simulink model "EX_opt_1_model"  (R2025b)
settings: Solver=ode4  StartTime=0.0  StopTime=T_SIMULATION  FixedStep=1e-3  RelTol=1e-3
values from neighbouring files (symbols this model uses):
  d = 0.165    [EX_opt_1.m]
  omega = 2    [EX_opt_1.m]    (also in EX_opt_2.m = zeros(size(t)))
  Q_INITIAL = [1;1;0]    [EX_opt_1.m]
  r = 0.03    [EX_opt_1.m]
  v = 0    [EX_opt_1.m]    (also in EX_opt_2.m = zeros(size(t)))
settings Model: Creator=llp  LastModifiedBy=llp

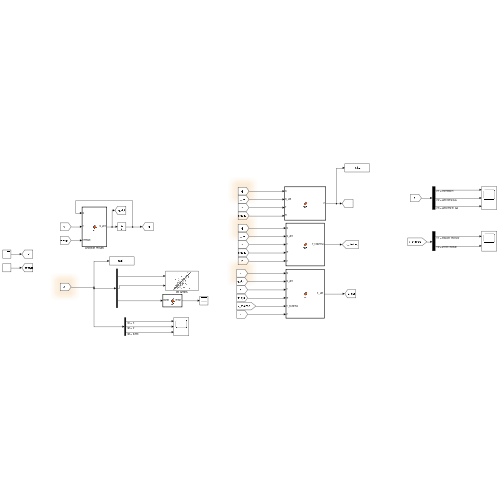
[thumbnail: Simulink's stored preview of the top-level diagram]
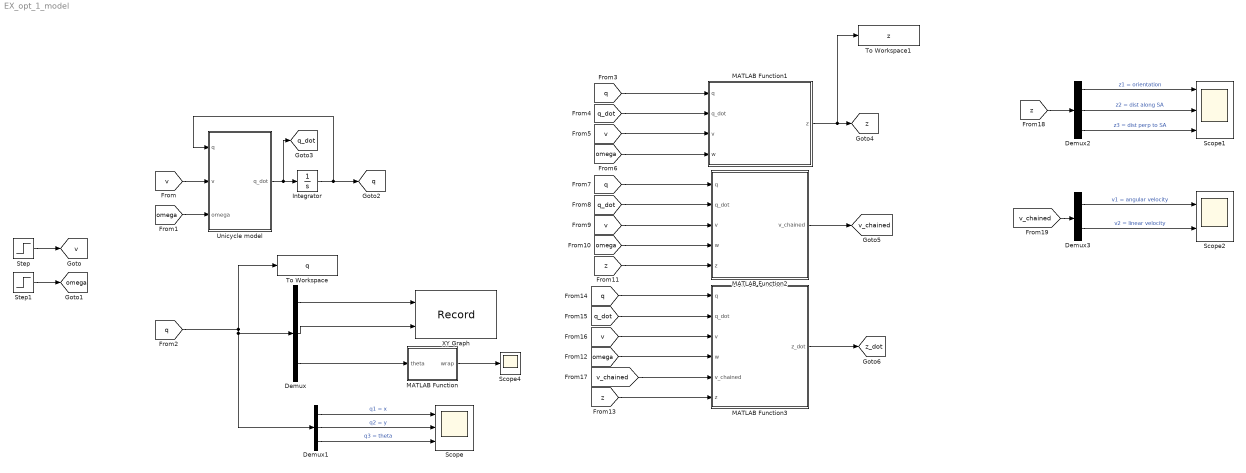
== system EX_opt_1_model ==
  Demux : Demux  Outputs=3
  Demux1 : Demux  Outputs=3
  Demux2 : Demux  Outputs=3
  Demux3 : Demux  Outputs=2
  Integrator : Integrator  InitialCondition=Q_INITIAL
  MATLAB Function : MATLAB Function  TreatAsAtomicUnit=on
  MATLAB Function1 : MATLAB Function  TreatAsAtomicUnit=on
  MATLAB Function2 : MATLAB Function  TreatAsAtomicUnit=on
  MATLAB Function3 : MATLAB Function  TreatAsAtomicUnit=on
  Scope : Scope  NumInputPorts=3
      settings: ActiveDisplayYMinimum=-4.1874997872268764  ActiveDisplayYMaximum=22.687499976358314
  Scope1 : Scope  NumInputPorts=3
      settings: ActiveDisplayYMinimum=-1  ActiveDisplayYMaximum=1
  Scope2 : Scope  NumInputPorts=2
      settings: ActiveDisplayYMinimum=-1  ActiveDisplayYMaximum=1  DataLoggingVariableName=ScopeData2
  Scope4 : Scope
      settings: ActiveDisplayYMinimum=-1.0000416736103395  ActiveDisplayYMaximum=-0.99962493750694481  DataLoggingVariableName=ScopeData4
  Step : Step  Time=0  After=v  SampleTime=0
  Step1 : Step  Time=0  After=omega  SampleTime=0
  To Workspace : ToWorkspace  VariableName=q  SaveFormat=Timeseries  SampleTime=-1
  To Workspace1 : ToWorkspace  VariableName=z  SaveFormat=Timeseries  SampleTime=-1
  Unicycle model : MATLAB Function  TreatAsAtomicUnit=on
  XY Graph : Record  NumPorts=2.0  FileSettingsInternal="{\"entries\":[{\"content\":{\"excelSettings\":{\"content\":{},\"type\":\"Streamout.ExcelSettings\"},\"parquetSettings\":{\"content\":{},\"type\":\"Streamout.ParquetSettings\"}},\"type\":\"Streamout.FileSettingStorage\",\"uuid\":\"\"}],\"packageUris\":[\"http:\\/\\/schema.mathworks.com\\/mf0\\/streamout_blocks\\/R2020a\"],\"version\":\"1.0\"}"  FrameSettings=[0, 0]  Layout=[1 1]  SignalsInternal="{\"entries\":[{\"content\":{\"signals\":[{\"content\":{\"blockPath\":[],\"dimensions\":[1,1],\"domain\":\"\",\"lineColor\":\"#a2142f\",\"plots\":[ 1 ],\"port\":1,\"sid\":[\"\"],\"signalID\":1,\"signalName\":\"Demux:1\"},\"type\":\"RecordBlkView.Signal\",\"uuid\":\"\"},{\"content\":{\"blockPath\":[],\"dimensions\":[1,1],\"domain\":\"\",\"lineColor\":\"#139fff\",\"plots\":[ 1 ],\"port\":2,\"sid\":[\"\"],\"signalID\":2,\"signalName\":\"Demux:2\"},\"type\":\"RecordBlkView.Signal\",\"uuid\":\"\"}]},\"type\":\"RecordBlkView.InputSignals\",\"uuid\":\"\"}],\"packageUris\":[\"http:\\/\\/schema.mathworks.com\\/mf0\\/streamout_blocks\\/R2020a\"],\"version\":\"1.0\"}"  VisualizationBindings="{\"xyplotplugin\":{\"info\":[{\"series\":[{\"bindingParametersList\":[{\"parameter\":\"X-Axis\",\"signalID\":1,\"signalName\":\"Demux:1\"},{\"parameter\":\"Y-Axis\",\"signalID\":2,\"signalName\":\"Demux:2\"}],\"seriesID\":0}],\"subplotID\":1}]}}"  CompatibilityTag=XY
  tag scope: omega=global, q=global, q_dot=global, v=global, v_chained=global, z=global, z_dot=global
  wires:
  Unicycle model/1(q_dot) -> [q_dot], Integrator/1
  Integrator/1 -> [q], Unicycle model/1(q)
  Step/1 -> [v]
  Step1/1 -> [omega]
  [v] -> Unicycle model/2(v)
  [omega] -> Unicycle model/3(omega)
  MATLAB Function/1(wrap) -> Scope4/1
  Demux1/1 -> Scope/1  "q1 = x"
  Demux/3 -> MATLAB Function/1(theta)
  Demux/2 -> XY Graph/2
  Demux/1 -> XY Graph/1
  Demux1/3 -> Scope/3  "q3 = theta"
  Demux1/2 -> Scope/2  "q2 = y"
  [q] -> To Workspace/1, Demux1/1, Demux/1
  [q] -> MATLAB Function1/1(q)
  [q_dot] -> MATLAB Function1/2(q_dot)
  [v] -> MATLAB Function1/3(v)
  [omega] -> MATLAB Function1/4(w)
  MATLAB Function1/1(z) -> To Workspace1/1, [z]
  [omega] -> MATLAB Function2/4(w)
  [v] -> MATLAB Function2/3(v)
  [q_dot] -> MATLAB Function2/2(q_dot)
  [q] -> MATLAB Function2/1(q)
  [z] -> MATLAB Function2/5(z)
  [q_dot] -> MATLAB Function3/2(q_dot)
  [z] -> MATLAB Function3/6(z)
  [v] -> MATLAB Function3/3(v)
  [q] -> MATLAB Function3/1(q)
  [omega] -> MATLAB Function3/4(w)
  MATLAB Function2/1(v_chained) -> [v_chained]
  [v_chained] -> MATLAB Function3/5(v_chained)
  MATLAB Function3/1(z_dot) -> [z_dot]
  [z] -> Demux2/1
  Demux2/1 -> Scope1/1  "z1 = orientation"
  Demux2/2 -> Scope1/2  "z2 = dist along SA"
  Demux2/3 -> Scope1/3  "z3 = dist perp to SA"
  [v_chained] -> Demux3/1
  Demux3/1 -> Scope2/1  "v1 = angular velocity"
  Demux3/2 -> Scope2/2  "v2 = linear velocity"

== matlab function EX_opt_1_model/Unicycle model ==
  data: q input; v input; q_dot output; omega input; r parameter; d parameter
function q_dot = fcn(q, v, omega, r, d)
%write the unicycle model
q_dot= zeros(3,1);

q_dot(1) = v*cos(q(3));
q_dot(2) = v*sin(q(3));
q_dot(3) = omega;

== matlab function EX_opt_1_model/MATLAB Function1 ==
  data: q input; z output; q_dot input; v input; w input
function z = fcn(q,q_dot,v,w)

z = zeros(3,1);
z(1)= q(3);
z(2)= q(1)*cos(q(3))+q(2)*sin(q(3));
z(3) = q(1)*sin(q(3))-q(2)*cos(q(3));

== matlab function EX_opt_1_model/MATLAB Function ==
  data: theta input; wrap output
function wrap = fcn(theta)

wrap = mod(theta+pi,2*pi)-pi ;

== matlab function EX_opt_1_model/MATLAB Function2 ==
  data: q input; v_chained output; q_dot input; v input; w input; z input
function v_chained = fcn(q,q_dot,v,w,z)


v_chained = zeros(2,1);
v_chained(1) = w;
v_chained(2) = v-z(3)*w;

== matlab function EX_opt_1_model/MATLAB Function3 ==
  data: q input; z_dot output; q_dot input; v input; w input; v_chained input; z input
function z_dot = fcn(q,q_dot,v,w,v_chained,z)


z_dot = zeros(3,1);
z_dot(1) = v_chained(1);
z_dot(2) = v_chained(2);
z_dot(3) = z(2)*v_chained(1);
